simulink model "modelo_motor_l1"  (R2018b)
settings: Solver=VariableStepAuto  StartTime=0.0  StopTime=t(end)  MaxStep=1e-3  RelTol=1e-3
undefined symbols (not defined in the file): I0, Km, Kp, Kw, pm
settings Model: Creator=19.00012-0  LastModifiedBy=19.00012-0

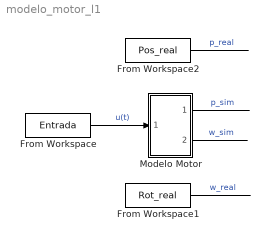
== system modelo_motor_l1 ==
  From Workspace : FromWorkspace  VariableName=Entrada  SampleTime=0
  From Workspace1 : FromWorkspace  VariableName=Rot_real  SampleTime=0
  From Workspace2 : FromWorkspace  VariableName=Pos_real  SampleTime=0
  Modelo Motor : Subsystem
  wires:
  From Workspace/1 -> Modelo Motor/1("u(t) ")  "u(t)"
  From Workspace2/1 -> ?  "p_real"
  Modelo Motor/1("Pos ") -> ?  "p_sim"
  Modelo Motor/2(Rot) -> ?  "w_sim"
  From Workspace1/1 -> ?  "w_real"

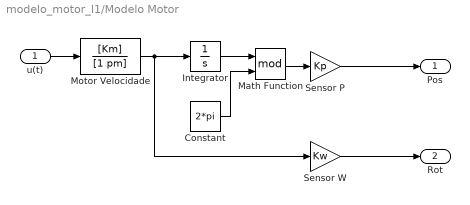
== system modelo_motor_l1/Modelo Motor ==
  "u(t) " : Inport
  Constant : Constant  Value=2*pi
  Integrator : Integrator  InitialCondition=I0
  Math Function : Math  Operator=mod  SaturateOnIntegerOverflow=on
  Motor Velocidade : TransferFcn  Numerator=[Km]  Denominator=[1 pm]
  Sensor P : Gain  Gain=Kp
  Sensor W : Gain  Gain=Kw
  "Pos " : Outport
  Rot : Outport  Port=2
  wires:
  "u(t) "/1 -> Motor Velocidade/1
  Sensor P/1 -> "Pos "/1
  Sensor W/1 -> Rot/1
  Motor Velocidade/1 -> Integrator/1, Sensor W/1
  Constant/1 -> Math Function/2
  Math Function/1 -> Sensor P/1
  Integrator/1 -> Math Function/1
